simulink model "PIDsim"  (R2016b)
settings: Solver=VariableStepAuto  StartTime=0.0  StopTime=2.5  FixedStep=.001  RelTol=1e-3
values from neighbouring files (symbols this model uses):
  A = 1.06    [PIDtest.m]
  d = 0    [PIDtest.m]
  dfreq = 10    [PIDtest.m]
  Kd = double(Kd)    [PIDmarginDesign.m]    (also in PIDtest.m = result(3))
  Ki = double(Ki)    [PIDmarginDesign.m]    (also in PIDtest.m = result(2); PImarginDesign.m)
  Kp = double(Kp)    [PIDmarginDesign.m]    (also in PIDtest.m = result(1); PImarginDesign.m)
  sensorrate = 1/10    (= 0.1)    [PIDtest.m]
  tau = 1.75    [PIDtest.m]
  td = .09    (= 0.09)    [PIDtest.m]
  v = .001    (= 0.001)    [PIDtest.m]
libraries: simulink x1
settings Model: Creator=chriskotcherha  LastModifiedBy=chriskotcherha
settings DataIOCC: SaveFormat=Array

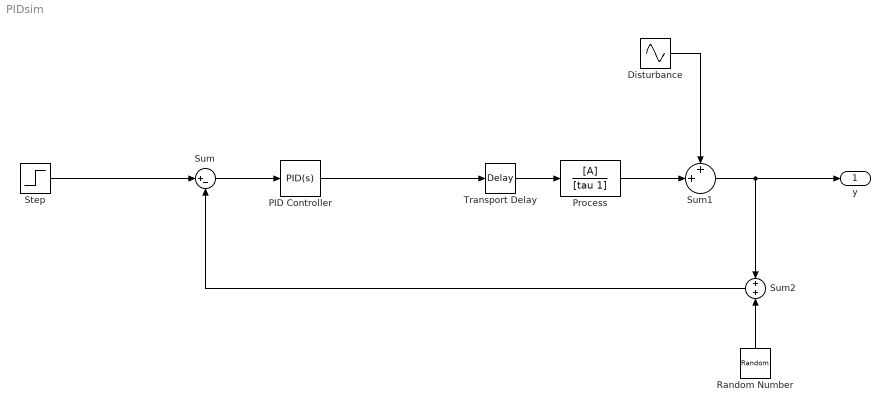
== system PIDsim ==
  Disturbance : Sin  Amplitude=d  Frequency=dfreq  SampleTime=0
  PID Controller : simulink/Continuous/PID Controller  Controller=PID  TimeDomain=Continuous-time  SampleTime=-1  IntegratorMethod=Forward Euler  FilterMethod=Forward Euler  Form=Parallel  UseFilter=on  ControllerParametersSource=internal  P=Kp  I=Ki  D=Kd  N=100  InitialConditionSource=internal  InitialConditionForIntegrator=0  InitialConditionForFilter=0  ExternalReset=none  LimitOutput=off  UpperSaturationLimit=inf  LowerSaturationLimit=-inf  LinearizeAsGain=on  AntiWindupMode=none  Kb=1  TrackingMode=off  Kt=1  PParamMin=[]  PParamMax=[]  IParamMin=[]  IParamMax=[]  DParamMin=[]  DParamMax=[]  NParamMin=[]  NParamMax=[]  KbParamMin=[]  KbParamMax=[]  KtParamMin=[]  KtParamMax=[]  POutMin=[]  POutMax=[]  IOutMin=[]  IOutMax=[]  DOutMin=[]  DOutMax=[]  NOutMin=[]  NOutMax=[]  KbOutMin=[]  KbOutMax=[]  KtOutMin=[]  KtOutMax=[]  IntegratorOutMin=[]  IntegratorOutMax=[]  FilterOutMin=[]  FilterOutMax=[]  SumOutMin=[]  SumOutMax=[]  SumI1OutMin=[]  SumI1OutMax=[]  SumI2OutMin=[]  SumI2OutMax=[]  SumI3OutMin=[]  SumI3OutMax=[]  SumDOutMin=[]  SumDOutMax=[]  SaturationOutMin=[]  SaturationOutMax=[]  IntegratorContinuousStateAttributes=''  IntegratorStateMustResolveToSignalObject=off  IntegratorRTWStateStorageClass=Auto  FilterContinuousStateAttributes=''  FilterStateMustResolveToSignalObject=off  FilterRTWStateStorageClass=Auto  DifferentiatorICPrevScaledInput=0  DifferentiatorOutMin=[]  DifferentiatorOutMax=[]
  Process : TransferFcn  Numerator=[A]  Denominator=[tau 1]
  Random Number : RandomNumber  Variance=v  SampleTime=sensorrate
  Step : Step  Time=0  SampleTime=0
  Sum : Sum  Inputs=|+-
  Sum1 : Sum  Inputs=++|
  Sum2 : Sum
  Transport Delay : TransportDelay  DelayTime=td
  y : Outport
  wires:
  Transport Delay/1 -> Process/1
  PID Controller/1 -> Transport Delay/1
  Step/1 -> Sum/1
  Sum/1 -> PID Controller/1
  Process/1 -> Sum1/2
  Disturbance/1 -> Sum1/1
  Sum1/1 -> y/1, Sum2/1
  Sum2/1 -> Sum/2
  Random Number/1 -> Sum2/2
